simulink model "uz_pmsm_model_9ph_21a"  (R2021a)
settings: Solver=FixedStepAuto  StartTime=0.0  StopTime=0.8  RelTol=1e-3
PreLoadFcn:
  | uz_pmsm_model_9ph_init_parameter
values from neighbouring files (symbols this model uses):
  c = 2/9*cat(1,tl1,tl2,tl3,tl4,tl5,tl6,tl7,tl8,tl9)    [uz_pmsm_model_9ph_init_parameter.m]
  friction_coefficient = 0.001    [uz_pmsm_model_9ph_init_parameter.m]
  inertia = 0.001    [uz_pmsm_model_9ph_init_parameter.m]
  k_i_d = 50    [uz_pmsm_model_9ph_init_parameter.m]
  k_i_q = 50    [uz_pmsm_model_9ph_init_parameter.m]
  k_p_d = 0.5    [uz_pmsm_model_9ph_init_parameter.m]
  k_p_q = 0.5    [uz_pmsm_model_9ph_init_parameter.m]
  L_d = 0.0023    [uz_pmsm_model_9ph_init_parameter.m]
  L_o1 = L_d/3    (= 0.000766666666667)    [uz_pmsm_model_9ph_init_parameter.m]
  L_o2 = L_d/3    (= 0.000766666666667)    [uz_pmsm_model_9ph_init_parameter.m]
  L_q = 0.0046    [uz_pmsm_model_9ph_init_parameter.m]
  L_x1 = L_d/3    (= 0.000766666666667)    [uz_pmsm_model_9ph_init_parameter.m]
  L_x2 = L_d/3    (= 0.000766666666667)    [uz_pmsm_model_9ph_init_parameter.m]
  L_y1 = L_d/3    (= 0.000766666666667)    [uz_pmsm_model_9ph_init_parameter.m]
  L_y2 = L_d/3    (= 0.000766666666667)    [uz_pmsm_model_9ph_init_parameter.m]
  L_zero = L_d/3    (= 0.000766666666667)    [uz_pmsm_model_9ph_init_parameter.m]
  polepair = 3    [uz_pmsm_model_9ph_init_parameter.m]
  psi_pm = 0.1028    [uz_pmsm_model_9ph_init_parameter.m]
  R_1 = 0.066    [uz_pmsm_model_9ph_init_parameter.m]
  static_friction_torque = 0.001    [uz_pmsm_model_9ph_init_parameter.m]
  ts = 2/1e6    (= 2e-06)    [uz_pmsm_model_9ph_init_parameter.m]
undefined symbols (not defined in the file or in its folder): Kpd, Tnd
libraries: pid_lib x3, simulink x2, spsAlphaBetaZerotodq0Lib x1, spsdq0toAlphaBetaZeroLib x1
(part 2 of 2)

== system uz_pmsm_model_9ph_21a/uz_pmsm_model_9ph/pmsm/integrator ==
  in : Inport
  reset : Inport  Port=2
  Delay1 : Delay  DelayLength=1  ExternalReset=Level
      settings: InputPortMap=u0,r5
  Gain : Gain  Gain=ts  OutDataTypeStr=Inherit: Same as input
  Sum3 : Sum  Inputs=|++  OutDataTypeStr=Inherit: Same as first input
  outt : Outport
  wires:
  reset/1 -> Delay1/2
  Gain/1 -> Sum3/1
  in/1 -> Gain/1
  Delay1/1 -> outt/1, Sum3/2
  Sum3/1 -> Delay1/1

== system uz_pmsm_model_9ph_21a/uz_pmsm_model_9ph/pmsm/integrator1 ==
  in : Inport
  reset : Inport  Port=2
  Delay1 : Delay  DelayLength=1  ExternalReset=Level
      settings: InputPortMap=u0,r5
  Gain : Gain  Gain=ts  OutDataTypeStr=Inherit: Same as input
  Sum3 : Sum  Inputs=|++  OutDataTypeStr=Inherit: Same as first input
  outt : Outport
  wires:
  reset/1 -> Delay1/2
  Gain/1 -> Sum3/1
  in/1 -> Gain/1
  Delay1/1 -> outt/1, Sum3/2
  Sum3/1 -> Delay1/1

== system uz_pmsm_model_9ph_21a/uz_pmsm_model_9ph/pmsm/integrator2 ==
  in : Inport
  reset : Inport  Port=2
  Delay1 : Delay  DelayLength=1  ExternalReset=Level
      settings: InputPortMap=u0,r5
  Gain : Gain  Gain=ts  OutDataTypeStr=Inherit: Same as input
  Sum3 : Sum  Inputs=|++  OutDataTypeStr=Inherit: Same as first input
  outt : Outport
  wires:
  reset/1 -> Delay1/2
  Gain/1 -> Sum3/1
  in/1 -> Gain/1
  Delay1/1 -> outt/1, Sum3/2
  Sum3/1 -> Delay1/1

== system uz_pmsm_model_9ph_21a/uz_pmsm_model_9ph/pmsm/integrator3 ==
  in : Inport
  reset : Inport  Port=2
  Delay1 : Delay  DelayLength=1  ExternalReset=Level
      settings: InputPortMap=u0,r5
  Gain : Gain  Gain=ts  OutDataTypeStr=Inherit: Same as input
  Sum3 : Sum  Inputs=|++  OutDataTypeStr=Inherit: Same as first input
  outt : Outport
  wires:
  reset/1 -> Delay1/2
  Gain/1 -> Sum3/1
  in/1 -> Gain/1
  Delay1/1 -> outt/1, Sum3/2
  Sum3/1 -> Delay1/1

== system uz_pmsm_model_9ph_21a/uz_pmsm_model_9ph/pmsm/integrator4 ==
  in : Inport
  reset : Inport  Port=2
  Delay1 : Delay  DelayLength=1  ExternalReset=Level
      settings: InputPortMap=u0,r5
  Gain : Gain  Gain=ts  OutDataTypeStr=Inherit: Same as input
  Sum3 : Sum  Inputs=|++  OutDataTypeStr=Inherit: Same as first input
  outt : Outport
  wires:
  reset/1 -> Delay1/2
  Gain/1 -> Sum3/1
  in/1 -> Gain/1
  Delay1/1 -> outt/1, Sum3/2
  Sum3/1 -> Delay1/1

== system uz_pmsm_model_9ph_21a/uz_pmsm_model_9ph/pmsm/integrator5 ==
  in : Inport
  reset : Inport  Port=2
  Delay1 : Delay  DelayLength=1  ExternalReset=Level
      settings: InputPortMap=u0,r5
  Gain : Gain  Gain=ts  OutDataTypeStr=Inherit: Same as input
  Sum3 : Sum  Inputs=|++  OutDataTypeStr=Inherit: Same as first input
  outt : Outport
  wires:
  reset/1 -> Delay1/2
  Gain/1 -> Sum3/1
  in/1 -> Gain/1
  Delay1/1 -> outt/1, Sum3/2
  Sum3/1 -> Delay1/1

== system uz_pmsm_model_9ph_21a/uz_pmsm_model_9ph/pmsm/integrator6 ==
  in : Inport
  reset : Inport  Port=2
  Delay1 : Delay  DelayLength=1  ExternalReset=Level
      settings: InputPortMap=u0,r5
  Gain : Gain  Gain=ts  OutDataTypeStr=Inherit: Same as input
  Sum3 : Sum  Inputs=|++  OutDataTypeStr=Inherit: Same as first input
  outt : Outport
  wires:
  reset/1 -> Delay1/2
  Gain/1 -> Sum3/1
  in/1 -> Gain/1
  Delay1/1 -> outt/1, Sum3/2
  Sum3/1 -> Delay1/1

== system uz_pmsm_model_9ph_21a/uz_pmsm_model_9ph/pmsm/integrator7 ==
  in : Inport
  reset : Inport  Port=2
  Delay1 : Delay  DelayLength=1  ExternalReset=Level
      settings: InputPortMap=u0,r5
  Gain : Gain  Gain=ts  OutDataTypeStr=Inherit: Same as input
  Sum3 : Sum  Inputs=|++  OutDataTypeStr=Inherit: Same as first input
  outt : Outport
  wires:
  reset/1 -> Delay1/2
  Gain/1 -> Sum3/1
  in/1 -> Gain/1
  Delay1/1 -> outt/1, Sum3/2
  Sum3/1 -> Delay1/1

== system uz_pmsm_model_9ph_21a/uz_pmsm_model_9ph/pmsm/integrator8 ==
  in : Inport
  reset : Inport  Port=2
  Delay1 : Delay  DelayLength=1  ExternalReset=Level
      settings: InputPortMap=u0,r5
  Gain : Gain  Gain=ts  OutDataTypeStr=Inherit: Same as input
  Sum3 : Sum  Inputs=|++  OutDataTypeStr=Inherit: Same as first input
  outt : Outport
  wires:
  reset/1 -> Delay1/2
  Gain/1 -> Sum3/1
  in/1 -> Gain/1
  Delay1/1 -> outt/1, Sum3/2
  Sum3/1 -> Delay1/1
